simulink model "hw1"  (R2016b)
settings: Solver=FixedStepAuto  StartTime=0.0  StopTime=10.0  FixedStep=0.001  RelTol=1e-3
settings Model: Creator=Franz  LastModifiedBy=Franz

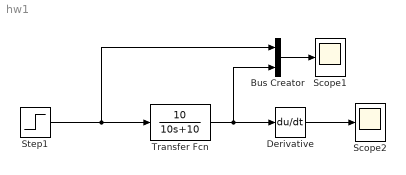
== system hw1 ==
  Bus Creator : BusCreator  Inputs=2
  Derivative : Derivative
  "Scope1 " : Scope
  "Scope2 " : Scope
  Step1 : Step  SampleTime=0
  Transfer Fcn : TransferFcn  Numerator=[10]  Denominator=[10 10]
  wires:
  Step1/1 -> Bus Creator/1, Transfer Fcn/1
  Transfer Fcn/1 -> Bus Creator/2, Derivative/1
  Derivative/1 -> "Scope2 "/1
  Bus Creator/1 -> "Scope1 "/1
